simulink model "biomasa2"  (R2016b)
settings: Solver=VariableStepAuto  StartTime=0.0  StopTime=10.0  RelTol=1e-3
settings Model: Creator=Asus  LastModifiedBy=Asus

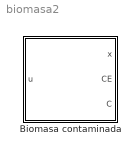
== system biomasa2 ==
  Biomasa contaminada : Subsystem  mask(Modelo){par=[0 0 0 0 0 0], x0=0}
      mask prompts: par "[r K  a  b  h  mu]"; x0 "Condiciones iniciales"
      mask help:
      | Modelo de concentración de contaminación en un ambiente
      | Entrada: contaminación
      | Salidas: biomasa de la población (x), concentración de toxina en el ambiente (Ce), cantidad de toxina en la biomasa de la población (C)
      mask init:
      | r = par(1); K = par(2); a = par(3); b = par(4); h = par(5); mu = par(6);
      mask Help: Los parámetros son positivos, mayores que cero.
      mask Display: image('D:\Dropbox\Ingeniería Matemática\Cuarto semestre\Monitoría lógica\imagen.jpg');

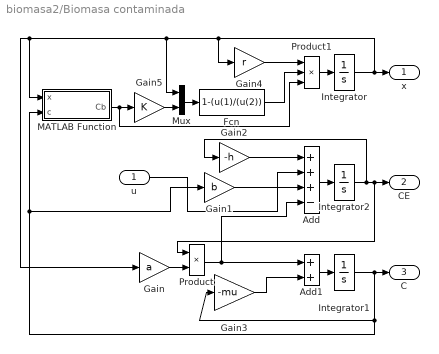
== system biomasa2/Biomasa contaminada ==
  u : Inport
  Add : Sum  Inputs=+++-
  Add1 : Sum
  Fcn : Fcn  Expr=1-(u(1)/(u(2))
  Gain : Gain  Gain=a
  Gain1 : Gain  Gain=b
  Gain2 : Gain  Gain=-h
  Gain3 : Gain  Gain=-mu
  Gain4 : Gain  Gain=r
  Gain5 : Gain  Gain=K
  Integrator : Integrator  InitialCondition=x0
  Integrator1 : Integrator  InitialCondition=x0
  Integrator2 : Integrator  InitialCondition=x0
  MATLAB Function : MATLAB Function  TreatAsAtomicUnit=on
  Mux : Mux  Inputs=2
  Product : Product
  Product1 : Product  Inputs=3
  x : Outport
  CE : Outport  Port=2
  C : Outport  Port=3
  wires:
  Product/1 -> Add/4, Add1/1
  Gain3/1 -> Add1/2
  Gain1/1 -> Add/3
  Gain4/1 -> Product1/1
  MATLAB Function/1(Cb) -> Product1/3, Gain5/1
  Product1/1 -> Integrator/1
  Integrator/1 -> Gain4/1, Mux/1, MATLAB Function/1(x), Gain/1, x/1
  Add1/1 -> Integrator1/1
  Integrator1/1 -> Gain3/1, Gain1/1, MATLAB Function/2(c), C/1
  Gain5/1 -> Mux/2
  Mux/1 -> Fcn/1
  Fcn/1 -> Product1/2
  u/1 -> Add/2
  Gain2/1 -> Add/1
  Add/1 -> Integrator2/1
  Integrator2/1 -> Gain2/1, Product/1, CE/1
  Gain/1 -> Product/2

== matlab function biomasa2/Biomasa contaminada/MATLAB Function ==
  data: x input; c input; Cb output
function Cb = fcn(x, c)
if x == 0
    Cb = 0;
else
    Cb = c/x;
end
end
